simulink subsystem "DAC"  (R2024b)
settings: Solver=VariableStepAuto  StartTime=0.0  StopTime=10.0  RelTol=1e-3
values from neighbouring files (symbols this model uses):
  Ts = 0.001    [Plant_ModelParameters.m]
undefined symbols (not defined in the file or in its folder): daq
settings Model: Creator=Riccardo Grosso  LastModifiedBy=Federico Bergami

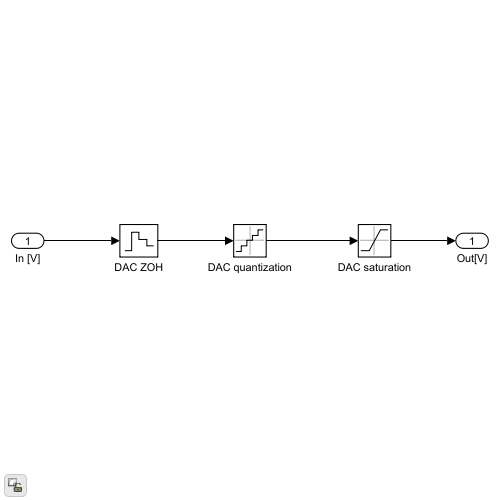
[thumbnail: Simulink's stored preview of the top-level diagram]
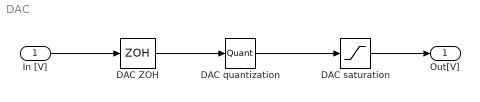
== system DAC ==
  In [V] : Inport
  DAC ZOH : ZeroOrderHold  SampleTime=Ts
  DAC quantization : Quantizer  QuantizationInterval=daq.dac.q
  DAC saturation : Saturate  UpperLimit=daq.dac.fs  LowerLimit=-daq.dac.fs  ZeroCross=off
  Out[V] : Outport  Unit=V
  wires:
  DAC quantization/1 -> DAC saturation/1
  DAC ZOH/1 -> DAC quantization/1
  In [V]/1 -> DAC ZOH/1
  DAC saturation/1 -> Out[V]/1
